simulink model "LSO"  (R2020b)
settings: Solver=VariableStepAuto  StartTime=0.0  StopTime=10.0  RelTol=1e-3
libraries: pid_lib x1
settings Model: Creator=jswl  LastModifiedBy=jswl
settings SFSimCC: CustomCodeUndefinedFunction=UseInterfaceOnly

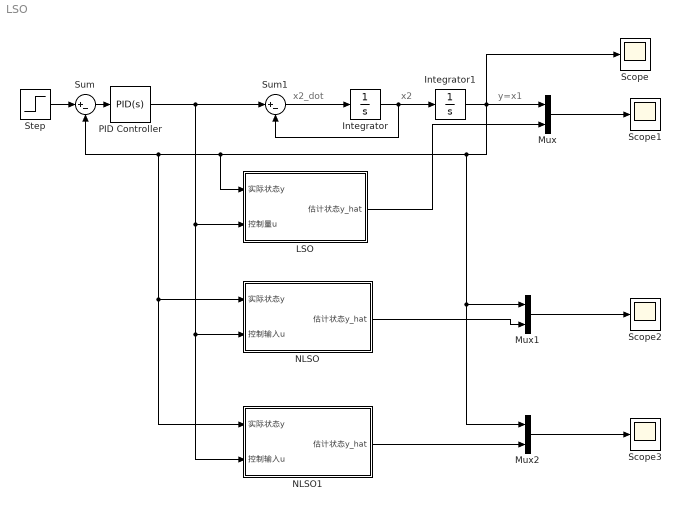
== system LSO ==
  note: y=x1
  note: x2
  note: x2_dot
  Integrator : Integrator  InitialCondition=0.1
  Integrator1 : Integrator  InitialCondition=0.1
  LSO : Subsystem
  Mux : Mux  Inputs=2
  Mux1 : Mux  Inputs=2
  Mux2 : Mux  Inputs=2
  NLSO : Subsystem
  NLSO1 : Subsystem
  PID Controller : pid_lib/PID Controller  Controller=PID  Form=Parallel  TimeDomain=Continuous-time  UseExternalTs=off  SampleTime=-1  IntegratorMethod=Forward Euler  FilterMethod=Forward Euler  ControllerParametersSource=internal  P=1  I=0.01  D=0  UseFilter=on  N=100  TunerSelectOption=Transfer Function Based (PID Tuner App)  InitialConditionSource=internal  InitialConditionForIntegrator=0  InitialConditionForFilter=0  DifferentiatorICPrevScaledInput=0  ExternalReset=none  TrackingMode=off  Kt=1  LimitOutput=off  SatLimitsSource=internal  UpperSaturationLimit=inf  LowerSaturationLimit=-inf  LinearizeAsGain=on  AntiWindupMode=none  Kb=1  POutMin=[]  POutMax=[]  IOutMin=[]  IOutMax=[]  DOutMin=[]  DOutMax=[]  NOutMin=[]  NOutMax=[]  SumOutMin=[]  SumOutMax=[]  SaturationOutMin=[]  SaturationOutMax=[]  PParamMin=[]  PParamMax=[]  IParamMin=[]  IParamMax=[]  DParamMin=[]  DParamMax=[]  NParamMin=[]  NParamMax=[]  KbParamMin=[]  KbParamMax=[]  KtParamMin=[]  KtParamMax=[]  KbOutMin=[]  KbOutMax=[]  KtOutMin=[]  KtOutMax=[]  IntegratorOutMin=[]  IntegratorOutMax=[]  FilterOutMin=[]  FilterOutMax=[]  SumI1OutMin=[]  SumI1OutMax=[]  SumI2OutMin=[]  SumI2OutMax=[]  SumI3OutMin=[]  SumI3OutMax=[]  SumI4OutMin=[]  SumI4OutMax=[]  SumDOutMin=[]  SumDOutMax=[]  DifferentiatorOutMin=[]  DifferentiatorOutMax=[]  FilterDiffOutCoefMin=[]  FilterDiffOutCoefMax=[]  ReciprocalOutMin=[]  ReciprocalOutMax=[]  SumDenOutMin=[]  SumDenOutMax=[]  SumNumOutMin=[]  SumNumOutMax=[]  DivideOutMin=[]  DivideOutMax=[]  UdiffTsProdOutMin=[]  UdiffTsProdOutMax=[]  NTsProdOutMin=[]  NTsProdOutMax=[]  UintegralTsProdOutMin=[]  UintegralTsProdOutMax=[]  UngainTsProdOutMin=[]  UngainTsProdOutMax=[]  IntegratorContinuousStateAttributes=''  IntegratorStateMustResolveToSignalObject=off  IntegratorRTWStateStorageClass=Auto  FilterContinuousStateAttributes=''  FilterStateMustResolveToSignalObject=off  FilterRTWStateStorageClass=Auto  ParallelPVariant=InternalParameters  IdealPVariant=Disabled  IVariant=InternalParameters  DVariant=InternalParameters  IntegratorVariant=Continuous  SatVariant=Disabled  AWVariant=Passthrough  PCopyVariant=Disabled  TRVariant=Disabled  FdbkBlocksVariant=Forward  IdealPFdbkVariant=Disabled  SatFdbkVariant=Disabled  DerivativeFilterVariant=ContFilter  NVariant=InternalParameters  NCopyVariant=Disabled  FilterICVariant=InternalICsFilter  IntegratorICVariant=InternalICs  ExternalResetVariant=Disabled  TRSumVariant=Passthrough  SumFdbkVariant=Disabled  SumVariant=Sum_PID  TsampFilterVariant=InternalTs  TsampNgainVariant=Passthrough  TsampIntegralVariant=Passthrough  ExternalSaturationOutDataTypeStr=Inherit: Same as second input
  Scope{,1..3} (4 alike) : Scope
  Step : Step  SampleTime=0
  Sum : Sum  Inputs=|+-
  Sum1 : Sum  Inputs=|+-
  wires:
  Sum/1 -> PID Controller/1
  Step/1 -> Sum/1
  Sum1/1 -> Integrator/1
  Integrator/1 -> Sum1/2, Integrator1/1
  Mux/1 -> Scope1/1
  LSO/1(估计状态y_hat) -> Mux/2
  Mux1/1 -> Scope2/1
  NLSO/1(估计状态y_hat) -> Mux1/2
  Integrator1/1 -> Mux/1, Mux2/1, Mux1/1, NLSO1/1(实际状态y), NLSO/1(实际状态y), Sum/2, LSO/1(实际状态y), Scope/1
  Mux2/1 -> Scope3/1
  NLSO1/1(估计状态y_hat) -> Mux2/2
  PID Controller/1 -> Sum1/1, NLSO1/2(控制输入u), NLSO/2(控制输入u), LSO/2(控制量u)

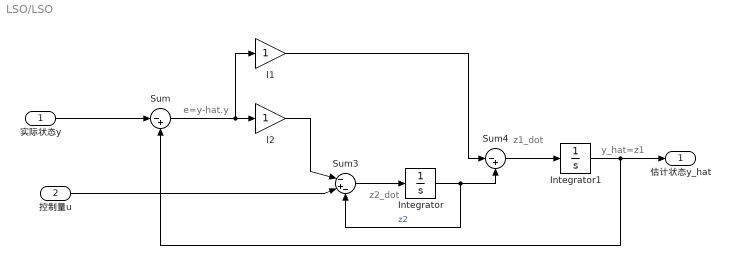
== system LSO/LSO ==
  note: z1_dot
  note: z2_dot
  note: y_hat=z1
  note: e=y-hat.y
  实际状态y : Inport
  控制量u : Inport  Port=2
  Integrator : Integrator
  Integrator1 : Integrator
  Sum : Sum  Inputs=|-+
  Sum3 : Sum  Inputs=|-+-
  Sum4 : Sum  Inputs=|-+
  l1 : Gain
  l2 : Gain
  估计状态y_hat : Outport  VectorParamsAs1DForOutWhenUnconnected=off
  wires:
  Integrator1/1 -> 估计状态y_hat/1, Sum/2
  Integrator/1 -> Sum3/3, Sum4/2  "z2"
  实际状态y/1 -> Sum/1
  Sum3/1 -> Integrator/1
  Sum4/1 -> Integrator1/1
  l2/1 -> Sum3/1
  Sum/1 -> l1/1, l2/1
  控制量u/1 -> Sum3/2
  l1/1 -> Sum4/1

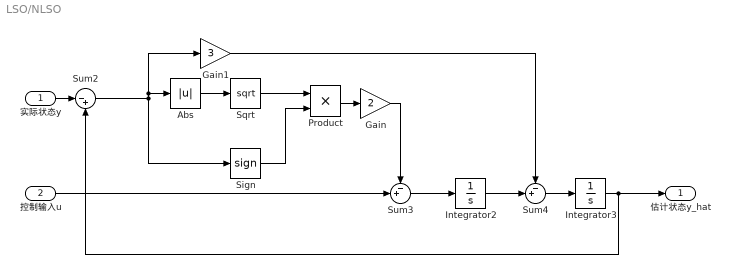
== system LSO/NLSO ==
  实际状态y : Inport
  控制输入u : Inport  Port=2
  Abs : Abs
  Gain : Gain  Gain=2
  Gain1 : Gain  Gain=3
  Integrator2 : Integrator
  Integrator3 : Integrator
  Product : Product
  Sign : Signum
  Sqrt : Sqrt  SaturateOnIntegerOverflow=on
  Sum2 : Sum  Inputs=|-+
  Sum3 : Sum  Inputs=-+|
  Sum4 : Sum  Inputs=-+|
  估计状态y_hat : Outport  VectorParamsAs1DForOutWhenUnconnected=off
  wires:
  Sum2/1 -> Gain1/1, Abs/1, Sign/1
  Product/1 -> Gain/1
  Sign/1 -> Product/2
  Integrator3/1 -> 估计状态y_hat/1, Sum2/2
  实际状态y/1 -> Sum2/1
  Sum4/1 -> Integrator3/1
  Integrator2/1 -> Sum4/2
  Abs/1 -> Sqrt/1
  Gain/1 -> Sum3/1
  Sqrt/1 -> Product/1
  Gain1/1 -> Sum4/1
  Sum3/1 -> Integrator2/1
  控制输入u/1 -> Sum3/2

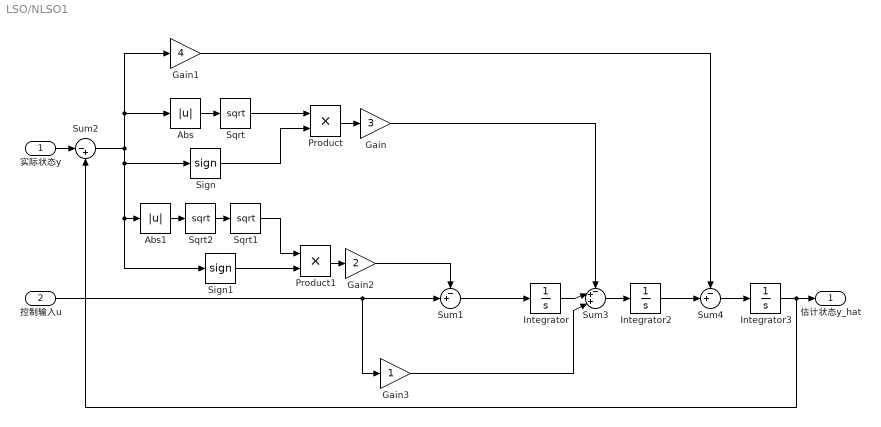
== system LSO/NLSO1 ==
  实际状态y : Inport
  控制输入u : Inport  Port=2
  Abs : Abs
  Abs1 : Abs
  Gain : Gain  Gain=3
  Gain1 : Gain  Gain=4
  Gain2 : Gain  Gain=2
  Gain3 : Gain
  Integrator : Integrator
  Integrator2 : Integrator
  Integrator3 : Integrator
  Product : Product
  Product1 : Product
  Sign : Signum
  Sign1 : Signum
  Sqrt : Sqrt  SaturateOnIntegerOverflow=on
  Sqrt1 : Sqrt  SaturateOnIntegerOverflow=on
  Sqrt2 : Sqrt  SaturateOnIntegerOverflow=on
  Sum1 : Sum  Inputs=-+|
  Sum2 : Sum  Inputs=|-+
  Sum3 : Sum  Inputs=-++|
  Sum4 : Sum  Inputs=-+|
  估计状态y_hat : Outport  VectorParamsAs1DForOutWhenUnconnected=off
  wires:
  Product/1 -> Gain/1
  Sign/1 -> Product/2
  Integrator3/1 -> 估计状态y_hat/1, Sum2/2
  实际状态y/1 -> Sum2/1
  Sum4/1 -> Integrator3/1
  Integrator2/1 -> Sum4/2
  Abs/1 -> Sqrt/1
  Gain/1 -> Sum3/1
  Sqrt/1 -> Product/1
  Gain1/1 -> Sum4/1
  Sum3/1 -> Integrator2/1
  Integrator/1 -> Sum3/2
  Abs1/1 -> Sqrt2/1
  Sum2/1 -> Abs/1, Gain1/1, Sign1/1, Abs1/1, Sign/1
  Sign1/1 -> Product1/2
  Sqrt1/1 -> Product1/1
  Sqrt2/1 -> Sqrt1/1
  Gain2/1 -> Sum1/1
  控制输入u/1 -> Gain3/1, Sum1/2
  Sum1/1 -> Integrator/1
  Product1/1 -> Gain2/1
  Gain3/1 -> Sum3/3
